simulink model "simulate_process"  (Simulink 10.2)
settings: Solver=VariableStepAuto  StartTime=0.0  StopTime=40  RelTol=1e-3  EnableMultiTasking=on
PreLoadFcn:
  | Left_figure = [0 0 0 0 0]
  | Right_figure = Left_figure
  | tout = 0
  | configure_lab
InitFcn:
  | configure_lab
StopFcn:
  | plot_figures
values from neighbouring files (symbols this model uses):
  lt = LinearTankModel    [PrepQuizScript.m]    (also in PrepQuizScript1.m; configure_lab.m; estimate_parameters.m)
  Ts = lt.SampleTime    [PrepQuizScript.m]    (also in PrepQuizScript1.m; configure_lab.m)
undefined symbols (not defined in the file or in its folder): CL_lqg_wn, Kff
libraries: mpclib x1
settings Model: Creator=his10eni  LastModifiedBy=johanl
settings DataIOCC: SaveFormat=Dataset  SignalLoggingSaveFormat=Dataset
settings DebuggingCC: UnderspecifiedInitializationDetection=Simplified  MergeDetectMultiDrivingBlocksExec=error  FcnCallInpInsideContextMsg=error  SFExecutionAtInitializationDiag=warning
settings HardwareCC: ProdBitPerPointer=64  ProdBitPerSizeT=64  ProdBitPerPtrDiffT=64  ProdLargestAtomicFloat=Float  ProdIntDivRoundTo=Zero  ProdEndianess=LittleEndian  ProdWordSize=64  ProdHWDeviceType=Intel->x86-64 (Windows64)
settings ModelReferenceCC: PropagateSignalLabelsOutOfModel=on
settings GRTTargetCC: CombineOutputUpdateFcns=on  GRTInterface=off

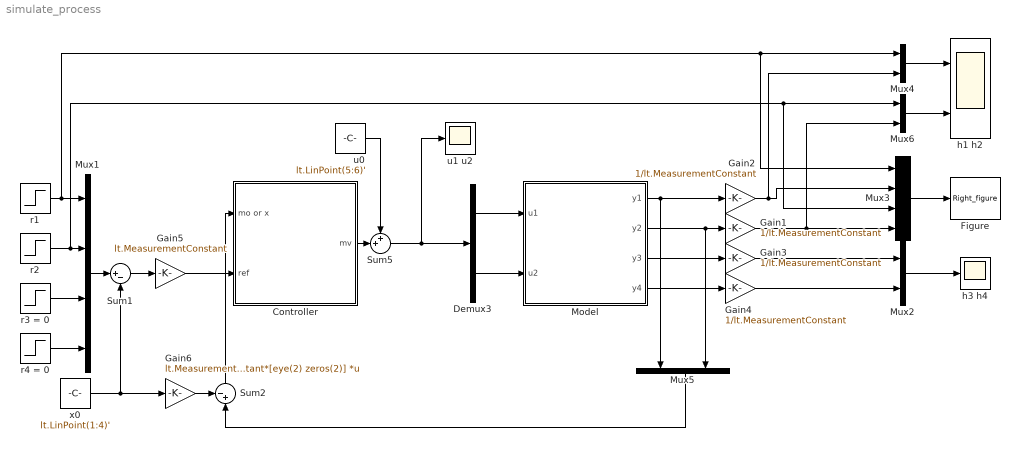
== system simulate_process ==
  "Controller " : Subsystem  Variant=on  VariantControlMode=label  VariantControl=Variant1  LabelModeActiveChoice=LQG
      mask Callback Control2: set_param(gcb,'LabelModeActiveChoice', 'LQG')
      mask Callback Control4: set_param(gcb,'LabelModeActiveChoice', 'KILL')
      mask Callback Control3: set_param(gcb,'LabelModeActiveChoice', 'MPC')
  Demux3 : Demux  Outputs=2
  "Figure " : ToWorkspace  VariableName=Right_figure  SampleTime=-1
      settings: Save2DSignal=2-D array (concatenate along first dimension)
      mask DialogControl Control2 Prompt: Left Figure
      mask DialogControl Control2 Callback: set_param(gcb,'VariableName', 'Left_figure')
      mask DialogControl Control2_copy Prompt: Right Figure
      mask DialogControl Control2_copy Callback: set_param(gcb,'VariableName', 'Right_figure')
  Gain{1..4} (4 alike) : Gain  Gain=1/lt.MeasurementConstant
  Gain5 : Gain  Gain=lt.MeasurementConstant
  Gain6 : Gain  Gain=lt.MeasurementConstant*[eye(2) zeros(2)]  Multiplication=Matrix(K*u)
  Model : Subsystem  Variant=on  VariantControlMode=label  VariantControl=Nonlinear  LabelModeActiveChoice=Nonlinear  PropagateVariantConditions=on
      mask Callback LinearButton:
      | %set_param(gcb, 'VariantControl', 'Linear')
      | set_param(gcb,'LabelModeActiveChoice', 'Linear')
      mask Callback NLbutton:
      | %set_param(gcb, 'VariantControl', 'Nonlinear')
      | set_param(gcb,'LabelModeActiveChoice', 'Nonlinear')
      mask Callback RealButton: set_param(gcb,'LabelModeActiveChoice', 'Real')
      mask Display:
      | p = get_param(gcb, 'LabelModeActiveChoice');
      | msg = '\n \n Doubleclick to toggle \n between models';
      | switch p
      |     case {'Linear'}
      |         disp(['Linear Model' msg])
      |     case {'Nonlinear'}
      |         disp(['Nonlinear Model' msg])
      |     case {'Real'}
      |         disp(['Real process' msg])
      |     otherwise
      |         disp('Error')
      | end
      | 
      | port_label('output',1,'y1')
      | port_label('output',2,'y2')
      | port_label('output',3,'y3')
      | port_label('output',4,'y4')
      | 
      | port_label('input',1,'u1')
      | port_label('input',2,'u2')
  Mux1 : Mux
  Mux{2,4..6} (4 alike) : Mux  Inputs=2
  Mux3 : Mux
  Sum1 : Sum  Inputs=|+-  InputSameDT=on  SaturateOnIntegerOverflow=on  OutDataTypeStr=Inherit: Same as first input
  Sum2 : Sum  Inputs=-+|  InputSameDT=on  SaturateOnIntegerOverflow=on  OutDataTypeStr=Inherit: Same as first input
  Sum5 : Sum  Inputs=++|  InputSameDT=on  SaturateOnIntegerOverflow=on  OutDataTypeStr=Inherit: Same as first input
  h1 h2 : Scope  NumInputPorts=2
  h3 h4 : Scope
  r1 : Step  Time=100  Before=10  After=12  SampleTime=Ts
  r2 : Step  Time=100  Before=10  After=8  SampleTime=Ts
  r3 = 0 : Step  Time=0  After=0  SampleTime=Ts  ZeroCross=off
  r4 = 0 : Step  Time=0  After=0  SampleTime=Ts  ZeroCross=off
  u0 : Constant  Value=lt.LinPoint(5:6)'
  u1 u2 : Scope
  x0 : Constant  Value=lt.LinPoint(1:4)'
  wires:
  Mux1/1 -> Sum1/1
  u0/1 -> Sum5/1
  Model/2(y2) -> Gain1/1, Mux5/2
  Mux2/1 -> h3 h4/1
  Model/3(y3) -> Gain3/1
  Model/4(y4) -> Gain4/1
  Sum1/1 -> Gain5/1
  Gain2/1 -> Mux4/2, Mux3/2
  Gain1/1 -> Mux6/2, Mux3/4
  Gain3/1 -> Mux2/1
  Gain4/1 -> Mux2/2
  Gain6/1 -> Sum2/1
  Sum2/1 -> "Controller "/1(mo or x)
  x0/1 -> Sum1/2, Gain6/1
  r3 = 0/1 -> Mux1/3
  r4 = 0/1 -> Mux1/4
  Gain5/1 -> "Controller "/2(ref)
  r2/1 -> Mux6/1, Mux3/3, Mux1/2
  r1/1 -> Mux4/1, Mux3/1, Mux1/1
  Model/1(y1) -> Gain2/1, Mux5/1
  Demux3/1 -> Model/1(u1)
  Sum5/1 -> Demux3/1, u1 u2/1
  Mux5/1 -> Sum2/2
  "Controller "/1(mv) -> Sum5/2
  Mux3/1 -> "Figure "/1
  Demux3/2 -> Model/2(u2)
  Mux6/1 -> h1 h2/2
  Mux4/1 -> h1 h2/1

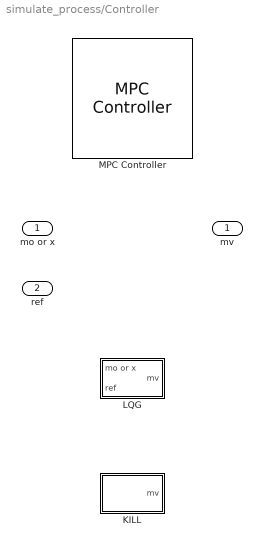
== system simulate_process/Controller  ==
  mo or x : Inport
  ref : Inport  Port=2
  KILL : Subsystem  VariantControl=KILL
  LQG : Subsystem  VariantControl=LQG
  "MPC Controller " : mpclib/MPC Controller  SCDEnableBlockLinearizationSpecification=on  VariantControl=MPC  mpcobj=mpcobj  is_multiple=0  enable_value=0  return_u0=off  updateMPCinCallerWorkspace=on  md_inport=off  mv_inport=off  uref_inport=off  return_cost=off  return_mvseq=off  return_qpstatus=off  return_xseq=off  return_state=off  return_ovseq=off  state_inport=off  umin_inport=off  umax_inport=off  ymin_inport=off  ymax_inport=off  cc_inport=off  ywt_inport=off  uwt_inport=off  duwt_inport=off  rhoeps_inport=off  pm_inport=off  MaximumP=10  HorizonChoice=FixedHorizon  n_ts=1  n_p=40  n_mv=2  n_md=0  n_ud=0  n_mo=2  n_uo=2  BlockDataType=double  SampleTimeInherited=off  switch_inport=off
  mv : Outport

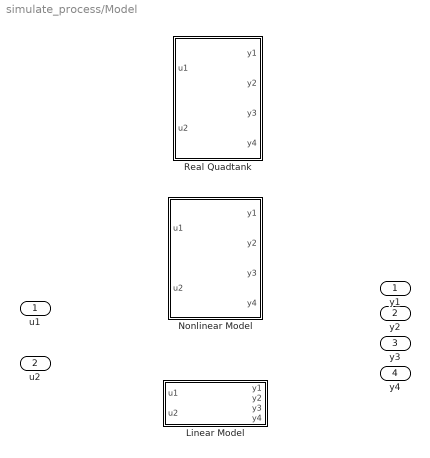
== system simulate_process/Model ==
  u1 : Inport
  u2 : Inport  Port=2
  "Linear Model " : Subsystem  VariantControl=Linear
  Nonlinear Model : Subsystem  VariantControl=Nonlinear
  Real Quadtank : Subsystem  AncestorBlock=tank/Real Quadtank  VariantControl=Real  mask{h=0.05}
  y1 : Outport
  y2 : Outport  Port=2
  y3 : Outport  Port=3
  y4 : Outport  Port=4

== system simulate_process/Controller /KILL ==
  Constant : Constant  Value=-lt.LinPoint(5:6)
  mv : Outport
  wires:
  Constant/1 -> mv/1

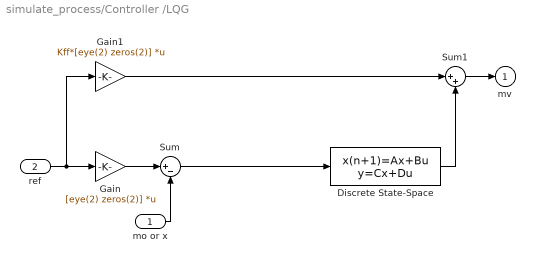
== system simulate_process/Controller /LQG ==
  mo or x : Inport
  ref : Inport  Port=2
  Discrete State-Space : DiscreteStateSpace  A=CL_lqg_wn.A  B=CL_lqg_wn.B  C=CL_lqg_wn.C  D=CL_lqg_wn.D  SampleTime=-1
  Gain : Gain  Gain=[eye(2) zeros(2)]  Multiplication=Matrix(K*u)
  Gain1 : Gain  Gain=Kff*[eye(2) zeros(2)]  Multiplication=Matrix(K*u)
  Sum : Sum  Inputs=|+-
  Sum1 : Sum  Inputs=|++
  mv : Outport
  wires:
  Discrete State-Space/1 -> Sum1/2
  mo or x/1 -> Sum/2
  ref/1 -> Gain1/1, Gain/1
  Gain/1 -> Sum/1
  Gain1/1 -> Sum1/1
  Sum1/1 -> mv/1
  Sum/1 -> Discrete State-Space/1

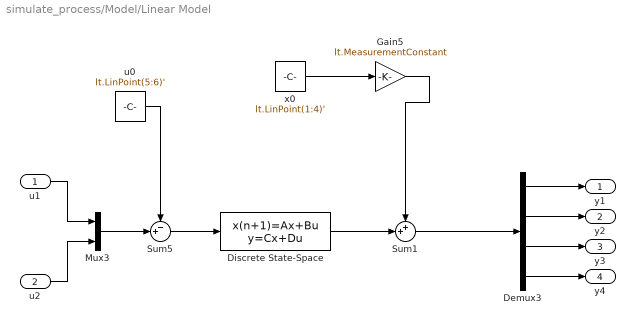
== system simulate_process/Model/Linear Model  ==
  u1 : Inport
  u2 : Inport  Port=2
  Demux3 : Demux
  Discrete State-Space : DiscreteStateSpace  A=lt.DtSys.A  B=lt.DtSys.B  C=lt.DtSys.C  D=lt.DtSys.D  InitialCondition=-lt.LinPoint(1:4)'  SampleTime=-1
  Gain5 : Gain  Gain=lt.MeasurementConstant
  Mux3 : Mux  Inputs=2
  Sum1 : Sum  Inputs=++|  InputSameDT=on  SaturateOnIntegerOverflow=on  OutDataTypeStr=Inherit: Same as first input
  Sum5 : Sum  Inputs=-+|  InputSameDT=on  SaturateOnIntegerOverflow=on  OutDataTypeStr=Inherit: Same as first input
  u0 : Constant  Value=lt.LinPoint(5:6)'
  x0 : Constant  Value=lt.LinPoint(1:4)'
  y1 : Outport
  y2 : Outport  Port=2
  y3 : Outport  Port=3
  y4 : Outport  Port=4
  wires:
  u1/1 -> Mux3/1
  u2/1 -> Mux3/2
  Demux3/1 -> y1/1
  Demux3/2 -> y2/1
  Demux3/3 -> y3/1
  Demux3/4 -> y4/1
  Mux3/1 -> Sum5/2
  u0/1 -> Sum5/1
  Sum5/1 -> Discrete State-Space/1
  Discrete State-Space/1 -> Sum1/2
  Sum1/1 -> Demux3/1
  x0/1 -> Gain5/1
  Gain5/1 -> Sum1/1

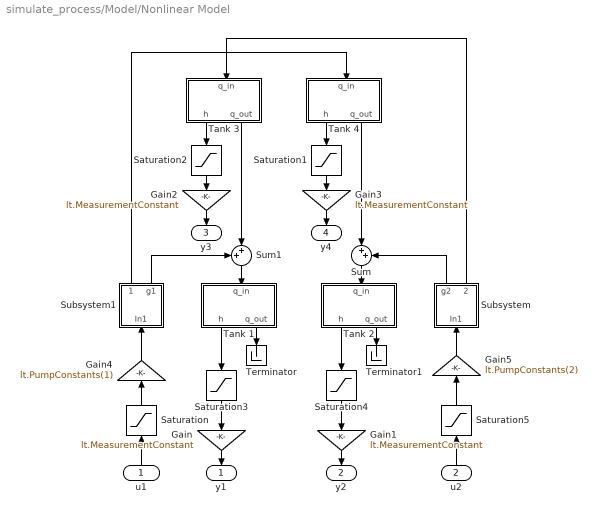
== system simulate_process/Model/Nonlinear Model ==
  u1 : Inport
  u2 : Inport  Port=2
  Gain{,1..3} (4 alike) : Gain  Gain=lt.MeasurementConstant
  Gain4 : Gain  Gain=lt.PumpConstants(1)
  Gain5 : Gain  Gain=lt.PumpConstants(2)
  Saturation : Saturate  UpperLimit=10  LowerLimit=0  LinearizeAsGain=off  ZeroCross=off
  Saturation{1..4} (4 alike) : Saturate  UpperLimit=16  LowerLimit=0  LinearizeAsGain=off  ZeroCross=off
  Saturation5 : Saturate  UpperLimit=10  LowerLimit=0  LinearizeAsGain=off  ZeroCross=off
  Subsystem : Subsystem
  Subsystem1 : Subsystem
  Sum : Sum  Inputs=|++
  Sum1 : Sum  Inputs=++|
  Tank 1 : Subsystem  mask{h0=eps, a=lt.OutletArea(1), A1=lt.TankArea(1), g=lt.Gravity}
      mask prompts: h0 "h0 [cm]"; a "a [cm^2]"; A1 "A [cm^2]"; g "g [cm/s^2]"
  Tank 2 : Subsystem  mask{h0=eps, a=lt.OutletArea(2), A1=lt.TankArea(2), g=lt.Gravity}
      mask prompts: h0 "h0 [cm]"; a "a [cm^2]"; A1 "A [cm^2]"; g "g [cm/s^2]"
  Tank 3 : Subsystem  mask{h0=eps, a=lt.OutletArea(3), A1=lt.TankArea(3), g=lt.Gravity}
      mask prompts: h0 "h0 [cm]"; a "a [cm^2]"; A1 "A [cm^2]"; g "g [cm/s^2]"
  Tank 4 : Subsystem  mask{h0=eps, a=lt.OutletArea(4), A1=lt.TankArea(4), g=lt.Gravity}
      mask prompts: h0 "h0 [cm]"; a "a [cm^2]"; A1 "A [cm^2]"; g "g [cm/s^2]"
  Terminator : Terminator
  Terminator1 : Terminator
  y1 : Outport
  y2 : Outport  Port=2
  y3 : Outport  Port=3
  y4 : Outport  Port=4
  wires:
  Gain/1 -> y1/1
  Tank 1/2(q_out) -> Terminator/1
  Tank 2/2(q_out) -> Terminator1/1
  Gain1/1 -> y2/1
  Gain2/1 -> y3/1
  Gain3/1 -> y4/1
  Sum/1 -> Tank 2/1(q_in)
  Tank 4/2(q_out) -> Sum/1
  Sum1/1 -> Tank 1/1(q_in)
  Tank 3/2(q_out) -> Sum1/2
  Subsystem/1(g2) -> Sum/2
  Subsystem1/2(g1) -> Sum1/1
  Subsystem/2(1-g2) -> Tank 3/1(q_in)
  Subsystem1/1(1-g1) -> Tank 4/1(q_in)
  Gain4/1 -> Subsystem1/1(In1)
  Gain5/1 -> Subsystem/1(In1)
  Tank 3/1(h) -> Saturation2/1
  Saturation2/1 -> Gain2/1
  Tank 4/1(h) -> Saturation1/1
  Saturation1/1 -> Gain3/1
  Saturation3/1 -> Gain/1
  Tank 1/1(h) -> Saturation3/1
  Saturation4/1 -> Gain1/1
  Tank 2/1(h) -> Saturation4/1
  u2/1 -> Saturation5/1
  Saturation5/1 -> Gain5/1
  Saturation/1 -> Gain4/1
  u1/1 -> Saturation/1

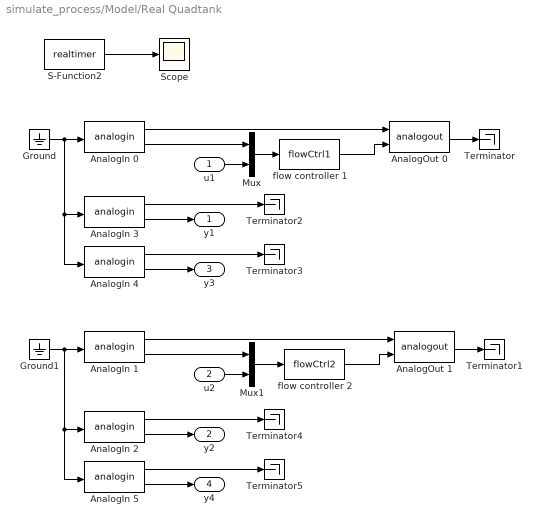
== system simulate_process/Model/Real Quadtank ==
  u1 : Inport
  u2 : Inport  Port=2
  AnalogIn 0 : S-Function  FunctionName=analogin  Parameters=h [35]  SFunctionDeploymentMode=off  EnableBusSupport=off
  AnalogIn 1 : S-Function  FunctionName=analogin  Parameters=h [34]  SFunctionDeploymentMode=off  EnableBusSupport=off
  AnalogIn 2 : S-Function  FunctionName=analogin  Parameters=h [33]  SFunctionDeploymentMode=off  EnableBusSupport=off
  AnalogIn 3 : S-Function  FunctionName=analogin  Parameters=h [31]  SFunctionDeploymentMode=off  EnableBusSupport=off
  AnalogIn 4 : S-Function  FunctionName=analogin  Parameters=h [30]  SFunctionDeploymentMode=off  EnableBusSupport=off
  AnalogIn 5 : S-Function  FunctionName=analogin  Parameters=h [32]  SFunctionDeploymentMode=off  EnableBusSupport=off
  AnalogOut 0 : S-Function  FunctionName=analogout  Parameters=h [31]  SFunctionDeploymentMode=off  EnableBusSupport=off
  AnalogOut 1 : S-Function  FunctionName=analogout  Parameters=h [30]  SFunctionDeploymentMode=off  EnableBusSupport=off
  Ground : Ground
  Ground1 : Ground
  Mux : Mux  Inputs=2
  Mux1 : Mux  Inputs=2
  S-Function2 : S-Function  FunctionName=realtimer  Parameters=h  SFunctionDeploymentMode=off  EnableBusSupport=off
  Scope : Scope
  Terminator{,1..5} (6 alike) : Terminator
  flow controller 1 : MATLABFcn  MATLABFcn=flowCtrl1  SampleTime=0.01
  flow controller 2 : MATLABFcn  MATLABFcn=flowCtrl2  SampleTime=0.01
  y1 : Outport
  y2 : Outport  Port=2
  y3 : Outport  Port=3
  y4 : Outport  Port=4
  wires:
  AnalogIn 0/2 -> Mux/1
  AnalogIn 1/2 -> Mux1/1
  flow controller 2/1 -> AnalogOut 1/2
  Mux1/1 -> flow controller 2/1
  u2/1 -> Mux1/2
  flow controller 1/1 -> AnalogOut 0/2
  Mux/1 -> flow controller 1/1
  u1/1 -> Mux/2
  AnalogIn 5/1 -> Terminator5/1
  AnalogIn 2/1 -> Terminator4/1
  Ground1/1 -> AnalogIn 1/1, AnalogIn 2/1, AnalogIn 5/1
  AnalogIn 5/2 -> y4/1
  AnalogIn 2/2 -> y2/1
  AnalogIn 4/1 -> Terminator3/1
  AnalogIn 3/1 -> Terminator2/1
  Ground/1 -> AnalogIn 4/1, AnalogIn 3/1, AnalogIn 0/1
  AnalogIn 4/2 -> y3/1
  AnalogIn 3/2 -> y1/1
  AnalogOut 1/1 -> Terminator1/1
  AnalogIn 1/1 -> AnalogOut 1/1
  AnalogOut 0/1 -> Terminator/1
  AnalogIn 0/1 -> AnalogOut 0/1
  S-Function2/1 -> Scope/1

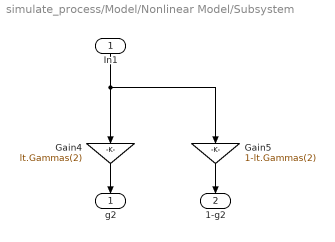
== system simulate_process/Model/Nonlinear Model/Subsystem ==
  In1 : Inport
  Gain4 : Gain  Gain=lt.Gammas(2)
  Gain5 : Gain  Gain=1-lt.Gammas(2)
  g2 : Outport
  1-g2 : Outport  Port=2
  wires:
  In1/1 -> Gain5/1, Gain4/1
  Gain4/1 -> g2/1
  Gain5/1 -> 1-g2/1

== system simulate_process/Model/Nonlinear Model/Subsystem1 ==
  In1 : Inport
  Gain4 : Gain  Gain=lt.Gammas(1)
  Gain5 : Gain  Gain=1-lt.Gammas(1)
  1-g1 : Outport
  g1 : Outport  Port=2
  wires:
  In1/1 -> Gain5/1, Gain4/1
  Gain5/1 -> 1-g1/1
  Gain4/1 -> g1/1

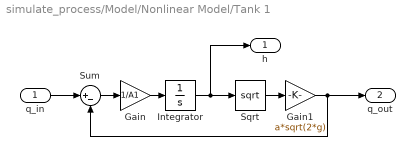
== system simulate_process/Model/Nonlinear Model/Tank 1 ==
  q_in : Inport
  Gain : Gain  Gain=1/A1
  Gain1 : Gain  Gain=a*sqrt(2*g)
  Integrator : Integrator  InitialCondition=h0  LimitOutput=on  UpperSaturationLimit=16  LowerSaturationLimit=eps
  Sqrt : Sqrt  SaturateOnIntegerOverflow=on
  Sum : Sum  Inputs=|+-
  h : Outport
  q_out : Outport  Port=2
  wires:
  Gain/1 -> Integrator/1
  Integrator/1 -> h/1, Sqrt/1
  Sum/1 -> Gain/1
  Gain1/1 -> q_out/1, Sum/2
  Sqrt/1 -> Gain1/1
  q_in/1 -> Sum/1

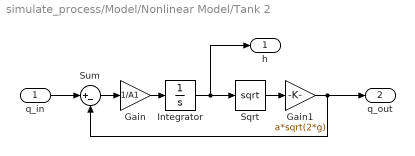
== system simulate_process/Model/Nonlinear Model/Tank 2 ==
  q_in : Inport
  Gain : Gain  Gain=1/A1
  Gain1 : Gain  Gain=a*sqrt(2*g)
  Integrator : Integrator  InitialCondition=h0  LimitOutput=on  UpperSaturationLimit=16  LowerSaturationLimit=eps
  Sqrt : Sqrt  SaturateOnIntegerOverflow=on
  Sum : Sum  Inputs=|+-
  h : Outport
  q_out : Outport  Port=2
  wires:
  Gain/1 -> Integrator/1
  Integrator/1 -> h/1, Sqrt/1
  Sum/1 -> Gain/1
  Gain1/1 -> q_out/1, Sum/2
  Sqrt/1 -> Gain1/1
  q_in/1 -> Sum/1

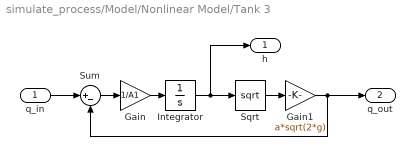
== system simulate_process/Model/Nonlinear Model/Tank 3 ==
  q_in : Inport
  Gain : Gain  Gain=1/A1
  Gain1 : Gain  Gain=a*sqrt(2*g)
  Integrator : Integrator  InitialCondition=h0  LimitOutput=on  UpperSaturationLimit=16  LowerSaturationLimit=eps
  Sqrt : Sqrt  SaturateOnIntegerOverflow=on
  Sum : Sum  Inputs=|+-
  h : Outport
  q_out : Outport  Port=2
  wires:
  Gain/1 -> Integrator/1
  Integrator/1 -> h/1, Sqrt/1
  Sum/1 -> Gain/1
  Gain1/1 -> q_out/1, Sum/2
  Sqrt/1 -> Gain1/1
  q_in/1 -> Sum/1

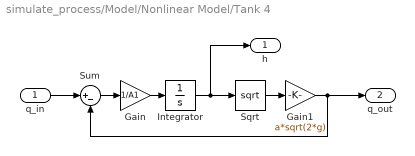
== system simulate_process/Model/Nonlinear Model/Tank 4 ==
  q_in : Inport
  Gain : Gain  Gain=1/A1
  Gain1 : Gain  Gain=a*sqrt(2*g)
  Integrator : Integrator  InitialCondition=h0  LimitOutput=on  UpperSaturationLimit=16  LowerSaturationLimit=eps
  Sqrt : Sqrt  SaturateOnIntegerOverflow=on
  Sum : Sum  Inputs=|+-
  h : Outport
  q_out : Outport  Port=2
  wires:
  Gain/1 -> Integrator/1
  Integrator/1 -> h/1, Sqrt/1
  Sum/1 -> Gain/1
  Gain1/1 -> q_out/1, Sum/2
  Sqrt/1 -> Gain1/1
  q_in/1 -> Sum/1
